simulink model "Zencar_rpo_2020_LQG_simModel_reactionWheel"  (R2020a)
settings: Solver=FixedStepAuto  StartTime=0.0  StopTime=40  FixedStep=1e-2  RelTol=1e-3
values from neighbouring files (symbols this model uses):
  A = a    [Zencar_rpo_2020_LQG_runScript_reactionWheel.m]    (also in Zencar_rpo_2020_LQG_simulationdata_reactionWheel.mat = [0  1  0; 21.2662842878  -0.985371341296  0.492685670648; -2)
  Ad = sysd.A    [Zencar_rpo_2020_LQG_runScript_reactionWheel.m]    (also in Zencar_rpo_2020_LQG_simulationdata_reactionWheel.mat = [1.00105829554  0.0099544956971  2.42643093775e-05; 0.211179)
  B = b    [Zencar_rpo_2020_LQG_runScript_reactionWheel.m]    (also in Zencar_rpo_2020_LQG_simulationdata_reactionWheel.mat = [0 -9.85371341296 72.353713413])
  Bd = sysd.B    [Zencar_rpo_2020_LQG_runScript_reactionWheel.m]    (also in Zencar_rpo_2020_LQG_simulationdata_reactionWheel.mat = [-0.00048528618755 -0.0963331348828 0.710167659151])
  bm = 0.05    [Zencar_rpo_2020_LQG_runScript_reactionWheel.m]    (also in Zencar_rpo_2020_LQG_simulationdata_reactionWheel.mat)
  bw = 0.1    [Zencar_rpo_2020_LQG_runScript_reactionWheel.m]    (also in Zencar_rpo_2020_LQG_simulationdata_reactionWheel.mat)
  C = c    [Zencar_rpo_2020_LQG_runScript_reactionWheel.m]    (also in Zencar_rpo_2020_LQG_simulationdata_reactionWheel.mat = [1  0  0; 0  1  0; 0  0  1])
  fi0 = -0.20    (= -0.2)    [Zencar_rpo_2020_LQG_runScript_reactionWheel.m]    (also in Zencar_rpo_2020_LQG_simulationdata_reactionWheel.mat)
  H = [1 0 0]    [Zencar_rpo_2020_LQG_runScript_reactionWheel.m]    (also in Zencar_rpo_2020_LQG_simulationdata_reactionWheel.mat)
  I = Imo+Iwo+Ibo    (= 0.101484583333)    [Zencar_rpo_2020_LQG_runScript_reactionWheel.m]    (also in Zencar_rpo_2020_LQG_simulationdata_reactionWheel.mat)
  Iw = mw*rw^2    (= 0.016)    [Zencar_rpo_2020_LQG_runScript_reactionWheel.m]    (also in Zencar_rpo_2020_LQG_simulationdata_reactionWheel.mat)
  K = k    [Zencar_rpo_2020_LQG_runScript_reactionWheel.m]    (also in Zencar_rpo_2020_LQG_simulationdata_reactionWheel.mat = [-13.1563542739 -3.87745747871 -0.104772255751])
  Kmgl = (mm*lm + mw*mw + mb*lb)*g    (= 2.1582)    [Zencar_rpo_2020_LQG_runScript_reactionWheel.m]    (also in Zencar_rpo_2020_LQG_simulationdata_reactionWheel.mat)
  P = zeros(3)    [Zencar_rpo_2020_LQG_runScript_reactionWheel.m]    (also in Zencar_rpo_2020_LQG_simulationdata_reactionWheel.mat = [0  0  0; 0  0  0; 0  0  0])
  V = 1*eye(3)    [Zencar_rpo_2020_LQG_runScript_reactionWheel.m]    (also in Zencar_rpo_2020_LQG_simulationdata_reactionWheel.mat = [1  0  0; 0  1  0; 0  0  1])
  W = 100    [Zencar_rpo_2020_LQG_runScript_reactionWheel.m]    (also in Zencar_rpo_2020_LQG_simulationdata_reactionWheel.mat)
  xhat = [fi0+(-1)^randi(10)*rand*2*pi/3200,0,0]'    [Zencar_rpo_2020_LQG_runScript_reactionWheel.m]    (also in Zencar_rpo_2020_LQG_simulationdata_reactionWheel.mat = [-0.200499281891 0 0])
undefined symbols (not defined in the file or in its folder): Continuous, Time
libraries: ctrlSharedLib x1
settings Model: Creator=Palo  LastModifiedBy=Palo
settings SolverCC: PositivePriorityOrder=on
settings DebuggingCC: InheritedTsInSrcMsg=none

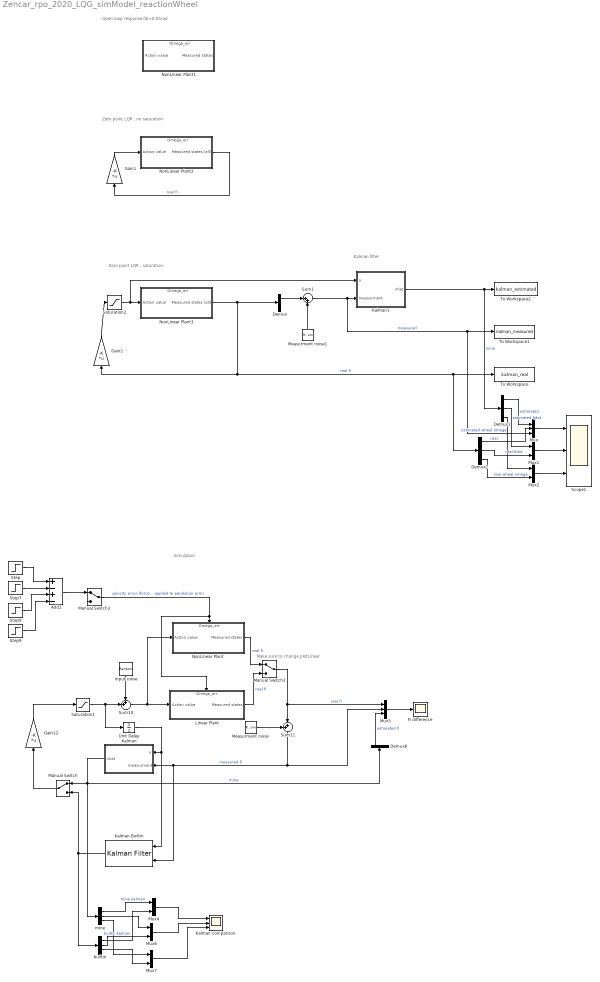
== system Zencar_rpo_2020_LQG_simModel_reactionWheel ==
  note: Open loop response fi0=0.05rad
  note: Zero point LQR , no saturation
  note: Zero point LQR , saturation
  note: Kalman filter
  note: Simulation
  note: Make sure to change plotLinear
  Add2 : Sum  Inputs=+-+-
  Demux{,1..2,6} (4 alike) : Demux  Outputs=3
  Fi difference : Scope
  Gain1 : Gain  Gain=-K  Multiplication=Matrix(K*u) (u vector)
  Gain12 : Gain  Gain=-K  Multiplication=Matrix(K*u) (u vector)
  Gain2 : Gain  Gain=-K  Multiplication=Matrix(K*u) (u vector)
  Input noise : RandomNumber  Variance=0.005  SampleTime=1e-2
  Kalman : Subsystem
  Kalman Builtin : ctrlSharedLib/Kalman Filter  TimeDomain=Continuous-Time  UseCurrentEstimator=on  ModelSource=Individual A, B, C, D matrices  ModelSourceVariable=sys  A=A  B=B  C=H  D=[0]  NumberOfStates=2  NumberOfInputs=2  NumberOfOutputs=2  InitialEstimateSource=Dialog  X0=xhat  P0=10  UseK=off  UseGH=off  NumberOfProcessNoiseInputs=2  G=1  TimeInvariantG=on  H=0  TimeInvariantH=on  Q=V  TimeInvariantQ=on  R=W  TimeInvariantR=on  N=0  TimeInvariantN=on  AddInputPort=on  AddEnablePort=off  OutputEstimatedY=off  OutputP=off  Ts=-1
  Kalman comparison : Scope  NumInputPorts=3
  Kalman1 : Subsystem
  Linear Plant : Subsystem
      settings: PortSchema="{\"entries\":[{\"content\":{\"sides\":[{\"content\":{\"connectorIds\":[\"In1\"]},\"type\":\"ConnectorPlacement.EquallySpacedRectSide\",\"uuid\":\"cef5a7e4-1169-406f-b141-8375d8af5010\"},{\"content\":{\"connectorIds\":[\"Out1\"],\"side\":\"RIGHT\"},\"type\":\"ConnectorPlacement.EquallySpacedRectSide\",\"uuid\":\"2cc08554-135f-4c1e-bb7d-3e74a7023c76\"},{\"content\":{\"connectorIds\":[\"In2\"],\"side\":\"TOP\"},\"type\":\"ConnectorPlacement.EquallySpacedRectSide\",\"uuid\":\"582a160d-15c5-42e8-87fa-6e353e2a7fa0\"}]},\"type\":\"ConnectorPlacement.EquallySpacedConnector\",\"uuid\":\"6957a99b-b85f-4d62-b482-e6d5ad956caf\"}],\"packageUris\":[\"http://schema.mathworks.com/mf0/Connector/19700101\"],\"version\":\"1.0\"}"
  Manual Switch : ManualSwitch
  Manual Switch2 : ManualSwitch
  Manual Switch3 : ManualSwitch
  Measurment noise : RandomNumber  Variance=2*pi/3200  SampleTime=1e-2
  Measurment noise1 : RandomNumber  Variance=2*pi/3200  SampleTime=1e-2
  Mux : Mux  Inputs=3
  Mux{1..2,4,6..7} (5 alike) : Mux  Inputs=2
  Mux5 : Mux  Inputs=3
  NonLinear Plant : Subsystem
      settings: PortSchema="{\"entries\":[{\"content\":{\"sides\":[{\"content\":{\"connectorIds\":[\"In1\"]},\"type\":\"ConnectorPlacement.EquallySpacedRectSide\",\"uuid\":\"cef5a7e4-1169-406f-b141-8375d8af5010\"},{\"content\":{\"connectorIds\":[\"Out1\"],\"side\":\"RIGHT\"},\"type\":\"ConnectorPlacement.EquallySpacedRectSide\",\"uuid\":\"2cc08554-135f-4c1e-bb7d-3e74a7023c76\"},{\"content\":{\"connectorIds\":[\"In2\"],\"side\":\"TOP\"},\"type\":\"ConnectorPlacement.EquallySpacedRectSide\",\"uuid\":\"582a160d-15c5-42e8-87fa-6e353e2a7fa0\"},{\"content\":{\"connectorIds\":[],\"side\":\"BOTTOM\"},\"type\":\"ConnectorPlacement.EquallySpacedRectSide\",\"uuid\":\"8b1cd8be-bae2-40ab-822a-6c2014c2b0d3\"}]},\"type\":\"ConnectorPlacement.EquallySpacedConnector\",\"uuid\":\"6957a99b-b85f-4d62-b482-e6d5ad956caf\"}],\"packageUris\":[\"http://schema.mathworks.com/mf0/Connector/19700101\"],\"version\":\"1.0\"}"
  NonLinear Plant1 : Subsystem
      settings: PortSchema="{\"entries\":[{\"content\":{\"sides\":[{\"content\":{\"connectorIds\":[\"In1\"]},\"type\":\"ConnectorPlacement.EquallySpacedRectSide\",\"uuid\":\"cef5a7e4-1169-406f-b141-8375d8af5010\"},{\"content\":{\"connectorIds\":[\"Out1\"],\"side\":\"RIGHT\"},\"type\":\"ConnectorPlacement.EquallySpacedRectSide\",\"uuid\":\"2cc08554-135f-4c1e-bb7d-3e74a7023c76\"},{\"content\":{\"connectorIds\":[\"In2\"],\"side\":\"TOP\"},\"type\":\"ConnectorPlacement.EquallySpacedRectSide\",\"uuid\":\"582a160d-15c5-42e8-87fa-6e353e2a7fa0\"},{\"content\":{\"connectorIds\":[],\"side\":\"BOTTOM\"},\"type\":\"ConnectorPlacement.EquallySpacedRectSide\",\"uuid\":\"8b1cd8be-bae2-40ab-822a-6c2014c2b0d3\"}]},\"type\":\"ConnectorPlacement.EquallySpacedConnector\",\"uuid\":\"6957a99b-b85f-4d62-b482-e6d5ad956caf\"}],\"packageUris\":[\"http://schema.mathworks.com/mf0/Connector/19700101\"],\"version\":\"1.0\"}"
  NonLinear Plant2 : Subsystem
      settings: PortSchema="{\"entries\":[{\"content\":{\"sides\":[{\"content\":{\"connectorIds\":[\"In1\"]},\"type\":\"ConnectorPlacement.EquallySpacedRectSide\",\"uuid\":\"cef5a7e4-1169-406f-b141-8375d8af5010\"},{\"content\":{\"connectorIds\":[\"Out1\"],\"side\":\"RIGHT\"},\"type\":\"ConnectorPlacement.EquallySpacedRectSide\",\"uuid\":\"2cc08554-135f-4c1e-bb7d-3e74a7023c76\"},{\"content\":{\"connectorIds\":[\"In2\"],\"side\":\"TOP\"},\"type\":\"ConnectorPlacement.EquallySpacedRectSide\",\"uuid\":\"582a160d-15c5-42e8-87fa-6e353e2a7fa0\"},{\"content\":{\"connectorIds\":[],\"side\":\"BOTTOM\"},\"type\":\"ConnectorPlacement.EquallySpacedRectSide\",\"uuid\":\"8b1cd8be-bae2-40ab-822a-6c2014c2b0d3\"}]},\"type\":\"ConnectorPlacement.EquallySpacedConnector\",\"uuid\":\"6957a99b-b85f-4d62-b482-e6d5ad956caf\"}],\"packageUris\":[\"http://schema.mathworks.com/mf0/Connector/19700101\"],\"version\":\"1.0\"}"
  NonLinear Plant3 : Subsystem
      settings: PortSchema="{\"entries\":[{\"content\":{\"sides\":[{\"content\":{\"connectorIds\":[\"In1\"]},\"type\":\"ConnectorPlacement.EquallySpacedRectSide\",\"uuid\":\"cef5a7e4-1169-406f-b141-8375d8af5010\"},{\"content\":{\"connectorIds\":[\"Out1\"],\"side\":\"RIGHT\"},\"type\":\"ConnectorPlacement.EquallySpacedRectSide\",\"uuid\":\"2cc08554-135f-4c1e-bb7d-3e74a7023c76\"},{\"content\":{\"connectorIds\":[\"In2\"],\"side\":\"TOP\"},\"type\":\"ConnectorPlacement.EquallySpacedRectSide\",\"uuid\":\"582a160d-15c5-42e8-87fa-6e353e2a7fa0\"},{\"content\":{\"connectorIds\":[],\"side\":\"BOTTOM\"},\"type\":\"ConnectorPlacement.EquallySpacedRectSide\",\"uuid\":\"8b1cd8be-bae2-40ab-822a-6c2014c2b0d3\"}]},\"type\":\"ConnectorPlacement.EquallySpacedConnector\",\"uuid\":\"6957a99b-b85f-4d62-b482-e6d5ad956caf\"}],\"packageUris\":[\"http://schema.mathworks.com/mf0/Connector/19700101\"],\"version\":\"1.0\"}"
  Saturation1 : Saturate  UpperLimit=0.8  LowerLimit=-0.8
  Saturation2 : Saturate  UpperLimit=0.8  LowerLimit=-0.8
  Scope1 : Scope  NumInputPorts=3
  Step : Step  Time=3  After=4  SampleTime=0
  Step7 : Step  Time=3.05  After=4  SampleTime=0
  Step8 : Step  Time=5.6  After=-4  SampleTime=0
  Step9 : Step  Time=5.65  After=-4  SampleTime=0
  Sum1 : Sum  Inputs=|++
  Sum10 : Sum  Inputs=++|
  Sum11 : Sum  Inputs=++|
  To Workspace : ToWorkspace  VariableName=kalman_real  SaveFormat=Structure With Time  SampleTime=-1
  To Workspace1 : ToWorkspace  VariableName=kalman_measured  SaveFormat=Structure With Time  SampleTime=-1
  To Workspace2 : ToWorkspace  VariableName=kalman_estimated  SaveFormat=Structure With Time  SampleTime=-1
  Unit Delay : UnitDelay  SampleTime=-1  HasFrameUpgradeWarning=on
  builtin : Demux  Outputs=3
  mine : Demux  Outputs=3
  wires:
  Mux5/1 -> Fi difference/1
  Saturation1/1 -> Unit Delay/1, Sum10/2
  Kalman/1(xhat) -> Demux6/1, Manual Switch/1, mine/1  "mine"
  Kalman Builtin/1 -> Manual Switch/2, builtin/1
  Sum11/1 -> Mux5/2, Kalman Builtin/2, Kalman/2(measurment)  "measured fi"
  Demux6/1 -> Mux5/3  "estimated fi"
  Linear Plant/1(Measured states) -> Manual Switch2/2  "real fi"
  NonLinear Plant/1(Measured states) -> Manual Switch2/1  "real fi"
  Manual Switch2/1 -> Mux5/1, Sum11/2  "real fi"
  Step/1 -> Add2/1
  Step7/1 -> Add2/2
  Step8/1 -> Add2/3
  Step9/1 -> Add2/4
  Manual Switch3/1 -> Linear Plant/2(Omega_err), NonLinear Plant/2(Omega_err)  "velocity error (force applied to pendulum arm)"
  Add2/1 -> Manual Switch3/1
  Sum10/1 -> NonLinear Plant/1(Action value), Linear Plant/1(Action value)
  mine/1 -> Mux4/1  "mine kalman"
  builtin/1 -> Mux4/2  "builtin kalman"
  mine/2 -> Mux6/1
  mine/3 -> Mux7/1
  builtin/2 -> Mux6/2
  builtin/3 -> Mux7/2
  Mux4/1 -> Kalman comparison/1
  Mux6/1 -> Kalman comparison/2
  Mux7/1 -> Kalman comparison/3
  Unit Delay/1 -> Kalman Builtin/1, Kalman/1(u)
  Gain12/1 -> Saturation1/1
  Manual Switch/1 -> Gain12/1
  NonLinear Plant2/1(Measured states (all)) -> Gain1/1  "real fi"
  Gain1/1 -> NonLinear Plant2/1(Action value)
  Measurment noise/1 -> Sum11/1
  Gain2/1 -> Saturation2/1
  NonLinear Plant3/1(Measured states (all)) -> Demux/1, Gain2/1, Demux2/1, To Workspace/1  "real fi"
  Saturation2/1 -> Kalman1/1(u), NonLinear Plant3/1(Action value)
  Measurment noise1/1 -> Sum1/2
  Demux/1 -> Sum1/1
  Sum1/1 -> To Workspace1/1, Mux/3, Kalman1/2(measurment)  "measured"
  Kalman1/1(xhat) -> Demux1/1, To Workspace2/1  "mine"
  Mux/1 -> Scope1/1
  Mux1/1 -> Scope1/2
  Mux2/1 -> Scope1/3
  Demux1/1 -> Mux/1  "estimated"
  Demux1/2 -> Mux1/1  "estimated fidot"
  Demux1/3 -> Mux2/1  "estimated wheel omega"
  Demux2/1 -> Mux/2  "real"
  Demux2/2 -> Mux1/2  "real fidot"
  Demux2/3 -> Mux2/2  "real wheel omega"
  Input noise/1 -> Sum10/1

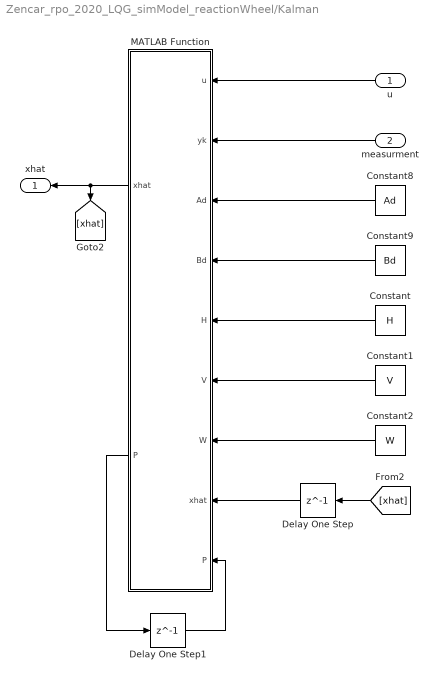
== system Zencar_rpo_2020_LQG_simModel_reactionWheel/Kalman ==
  u : Inport
  measurment : Inport  Port=2
  Constant : Constant  Value=H  VectorParams1D=off
  Constant1 : Constant  Value=V  VectorParams1D=off
  Constant2 : Constant  Value=W  VectorParams1D=off
  Constant8 : Constant  Value=Ad  VectorParams1D=off
  Constant9 : Constant  Value=Bd  VectorParams1D=off
  Delay One Step : Delay  DelayLength=1  InitialCondition=xhat
  Delay One Step1 : Delay  DelayLength=1  InitialCondition=P
  MATLAB Function : MATLAB Function  TreatAsAtomicUnit=on
  xhat : Outport
  wires:
  Delay One Step/1 -> MATLAB Function/8("xhat ")
  MATLAB Function/1(xhat) -> xhat/1, [xhat]
  MATLAB Function/2(P) -> Delay One Step1/1
  [xhat] -> Delay One Step/1
  measurment/1 -> MATLAB Function/2(yk)
  u/1 -> MATLAB Function/1(u)
  Delay One Step1/1 -> MATLAB Function/9("P ")
  Constant2/1 -> MATLAB Function/7(W)
  Constant1/1 -> MATLAB Function/6(V)
  Constant/1 -> MATLAB Function/5(H)
  Constant9/1 -> MATLAB Function/4(Bd)
  Constant8/1 -> MATLAB Function/3(Ad)

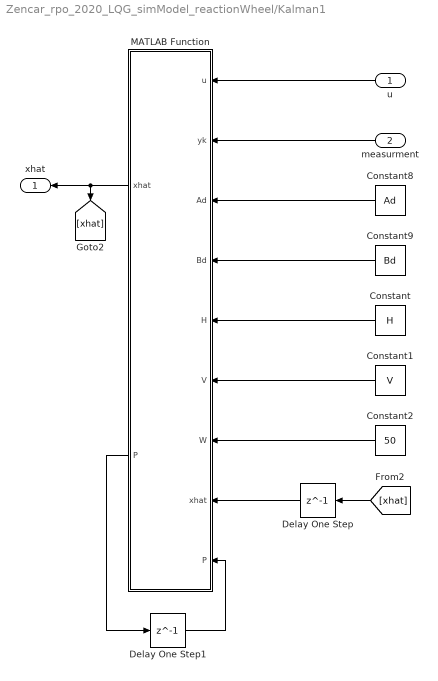
== system Zencar_rpo_2020_LQG_simModel_reactionWheel/Kalman1 ==
  u : Inport
  measurment : Inport  Port=2
  Constant : Constant  Value=H  VectorParams1D=off
  Constant1 : Constant  Value=V  VectorParams1D=off
  Constant2 : Constant  Value=50  VectorParams1D=off
  Constant8 : Constant  Value=Ad  VectorParams1D=off
  Constant9 : Constant  Value=Bd  VectorParams1D=off
  Delay One Step : Delay  DelayLength=1  InitialCondition=[0.2,0,0]'
  Delay One Step1 : Delay  DelayLength=1  InitialCondition=P
  MATLAB Function : MATLAB Function  TreatAsAtomicUnit=on
  xhat : Outport
  wires:
  Constant8/1 -> MATLAB Function/3(Ad)
  Constant9/1 -> MATLAB Function/4(Bd)
  Constant/1 -> MATLAB Function/5(H)
  Constant1/1 -> MATLAB Function/6(V)
  Constant2/1 -> MATLAB Function/7(W)
  Delay One Step1/1 -> MATLAB Function/9("P ")
  u/1 -> MATLAB Function/1(u)
  measurment/1 -> MATLAB Function/2(yk)
  [xhat] -> Delay One Step/1
  MATLAB Function/2(P) -> Delay One Step1/1
  MATLAB Function/1(xhat) -> [xhat], xhat/1
  Delay One Step/1 -> MATLAB Function/8("xhat ")

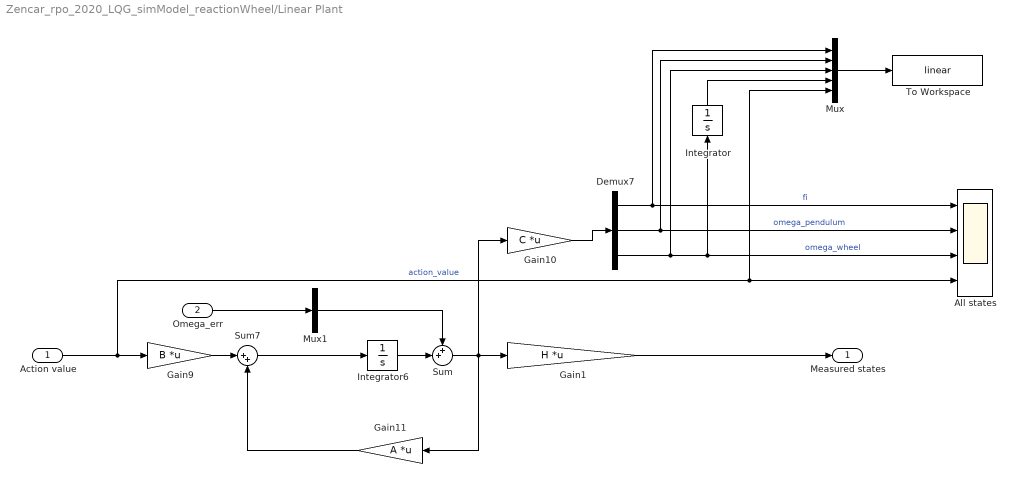
== system Zencar_rpo_2020_LQG_simModel_reactionWheel/Linear Plant ==
  Action value : Inport
  Omega_err : Inport  Port=2
  All states : Scope  NumInputPorts=4
  Demux7 : Demux  Outputs=3
  Gain1 : Gain  Gain=H  Multiplication=Matrix(K*u) (u vector)
  Gain10 : Gain  Gain=C  Multiplication=Matrix(K*u) (u vector)
  Gain11 : Gain  Gain=A  Multiplication=Matrix(K*u) (u vector)
  Gain9 : Gain  Gain=B  Multiplication=Matrix(K*u) (u vector)
  Integrator : Integrator
  Integrator6 : Integrator  InitialCondition=[fi0;0;0]
  Mux : Mux  Inputs=5
  Mux1 : Mux  Inputs=3
  Sum : Sum  Inputs=++|
  Sum7 : Sum  Inputs=|++
  To Workspace : ToWorkspace  VariableName=linear  SaveFormat=Structure With Time  SampleTime=-1
  Measured states : Outport
  wires:
  Gain9/1 -> Sum7/1
  Demux7/2 -> Mux/2, All states/2  "omega_pendulum"
  Demux7/3 -> Mux/3, Integrator/1, All states/3  "omega_wheel"
  Demux7/1 -> Mux/1, All states/1  "fi"
  Gain10/1 -> Demux7/1
  Gain11/1 -> Sum7/2
  Sum7/1 -> Integrator6/1
  Gain1/1 -> Measured states/1
  Action value/1 -> Mux/5, All states/4, Gain9/1  "action_value"
  Mux/1 -> To Workspace/1
  Integrator/1 -> Mux/4
  Omega_err/1 -> Mux1/2
  Mux1/1 -> Sum/1
  Integrator6/1 -> Sum/2
  Sum/1 -> Gain10/1, Gain11/1, Gain1/1

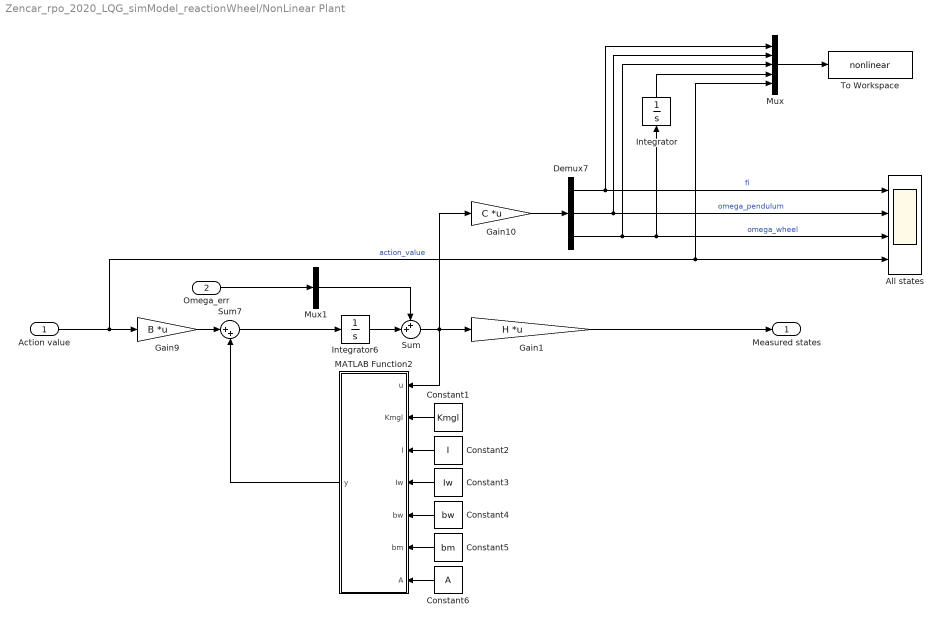
== system Zencar_rpo_2020_LQG_simModel_reactionWheel/NonLinear Plant ==
  Action value : Inport
  Omega_err : Inport  Port=2
  All states : Scope  NumInputPorts=4
  Constant1 : Constant  Value=Kmgl
  Constant2 : Constant  Value=I
  Constant3 : Constant  Value=Iw
  Constant4 : Constant  Value=bw
  Constant5 : Constant  Value=bm
  Constant6 : Constant  Value=A
  Demux7 : Demux  Outputs=3
  Gain1 : Gain  Gain=H  Multiplication=Matrix(K*u) (u vector)
  Gain10 : Gain  Gain=C  Multiplication=Matrix(K*u) (u vector)
  Gain9 : Gain  Gain=B  Multiplication=Matrix(K*u) (u vector)
  Integrator : Integrator
  Integrator6 : Integrator  InitialCondition=[fi0;0;0]
  MATLAB Function2 : MATLAB Function  TreatAsAtomicUnit=on
  Mux : Mux  Inputs=5
  Mux1 : Mux  Inputs=3
  Sum : Sum  Inputs=++|
  Sum7 : Sum  Inputs=|++
  To Workspace : ToWorkspace  VariableName=nonlinear  SaveFormat=Structure With Time  SampleTime=-1
  Measured states : Outport
  wires:
  Gain9/1 -> Sum7/1
  Demux7/2 -> Mux/2, All states/2  "omega_pendulum"
  Demux7/3 -> Mux/3, Integrator/1, All states/3  "omega_wheel"
  Demux7/1 -> Mux/1, All states/1  "fi"
  Gain10/1 -> Demux7/1
  Sum7/1 -> Integrator6/1
  Action value/1 -> Mux/5, All states/4, Gain9/1  "action_value"
  Mux/1 -> To Workspace/1
  Integrator/1 -> Mux/4
  Constant4/1 -> MATLAB Function2/5(bw)
  Constant3/1 -> MATLAB Function2/4(Iw)
  Constant5/1 -> MATLAB Function2/6(bm)
  Constant1/1 -> MATLAB Function2/2(Kmgl)
  MATLAB Function2/1(y) -> Sum7/2
  Constant2/1 -> MATLAB Function2/3(I)
  Integrator6/1 -> Sum/2
  Sum/1 -> Gain10/1, MATLAB Function2/1(u), Gain1/1
  Mux1/1 -> Sum/1
  Omega_err/1 -> Mux1/2
  Gain1/1 -> Measured states/1
  Constant6/1 -> MATLAB Function2/7(A)

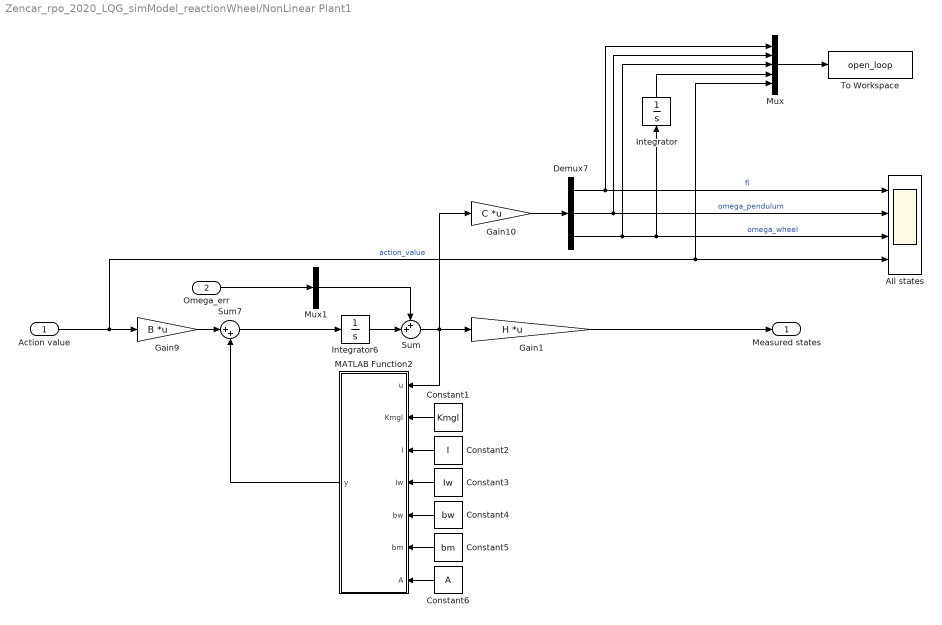
== system Zencar_rpo_2020_LQG_simModel_reactionWheel/NonLinear Plant1 ==
  Action value : Inport
  Omega_err : Inport  Port=2
  All states : Scope  NumInputPorts=4
  Constant1 : Constant  Value=Kmgl
  Constant2 : Constant  Value=I
  Constant3 : Constant  Value=Iw
  Constant4 : Constant  Value=bw
  Constant5 : Constant  Value=bm
  Constant6 : Constant  Value=A
  Demux7 : Demux  Outputs=3
  Gain1 : Gain  Gain=H  Multiplication=Matrix(K*u) (u vector)
  Gain10 : Gain  Gain=C  Multiplication=Matrix(K*u) (u vector)
  Gain9 : Gain  Gain=B  Multiplication=Matrix(K*u) (u vector)
  Integrator : Integrator
  Integrator6 : Integrator  InitialCondition=[0.05;0;0]
  MATLAB Function2 : MATLAB Function  TreatAsAtomicUnit=on
  Mux : Mux  Inputs=5
  Mux1 : Mux  Inputs=3
  Sum : Sum  Inputs=++|
  Sum7 : Sum  Inputs=|++
  To Workspace : ToWorkspace  VariableName=open_loop  SaveFormat=Structure With Time  SampleTime=-1
  Measured states : Outport
  wires:
  Constant6/1 -> MATLAB Function2/7(A)
  Gain1/1 -> Measured states/1
  Omega_err/1 -> Mux1/2
  Mux1/1 -> Sum/1
  Sum/1 -> Gain1/1, MATLAB Function2/1(u), Gain10/1
  Integrator6/1 -> Sum/2
  Constant2/1 -> MATLAB Function2/3(I)
  MATLAB Function2/1(y) -> Sum7/2
  Constant1/1 -> MATLAB Function2/2(Kmgl)
  Constant5/1 -> MATLAB Function2/6(bm)
  Constant3/1 -> MATLAB Function2/4(Iw)
  Constant4/1 -> MATLAB Function2/5(bw)
  Integrator/1 -> Mux/4
  Mux/1 -> To Workspace/1
  Action value/1 -> Gain9/1, All states/4, Mux/5  "action_value"
  Sum7/1 -> Integrator6/1
  Gain10/1 -> Demux7/1
  Demux7/1 -> All states/1, Mux/1  "fi"
  Demux7/3 -> All states/3, Integrator/1, Mux/3  "omega_wheel"
  Demux7/2 -> All states/2, Mux/2  "omega_pendulum"
  Gain9/1 -> Sum7/1

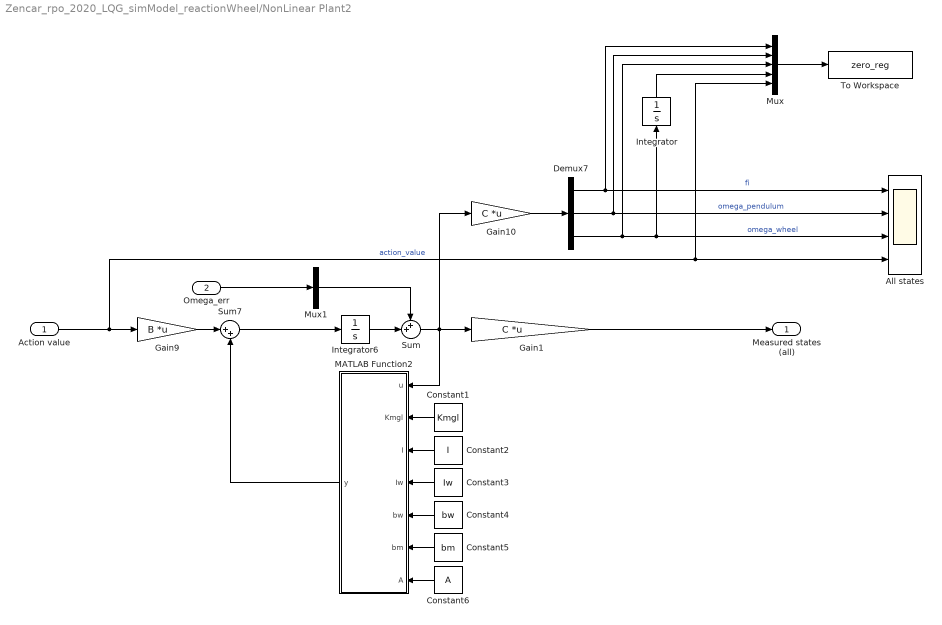
== system Zencar_rpo_2020_LQG_simModel_reactionWheel/NonLinear Plant2 ==
  Action value : Inport
  Omega_err : Inport  Port=2
  All states : Scope  NumInputPorts=4
  Constant1 : Constant  Value=Kmgl
  Constant2 : Constant  Value=I
  Constant3 : Constant  Value=Iw
  Constant4 : Constant  Value=bw
  Constant5 : Constant  Value=bm
  Constant6 : Constant  Value=A
  Demux7 : Demux  Outputs=3
  Gain1 : Gain  Gain=C  Multiplication=Matrix(K*u) (u vector)
  Gain10 : Gain  Gain=C  Multiplication=Matrix(K*u) (u vector)
  Gain9 : Gain  Gain=B  Multiplication=Matrix(K*u) (u vector)
  Integrator : Integrator
  Integrator6 : Integrator  InitialCondition=[-0.2;0;0]
  MATLAB Function2 : MATLAB Function  TreatAsAtomicUnit=on
  Mux : Mux  Inputs=5
  Mux1 : Mux  Inputs=3
  Sum : Sum  Inputs=++|
  Sum7 : Sum  Inputs=|++
  To Workspace : ToWorkspace  VariableName=zero_reg  SaveFormat=Structure With Time  SampleTime=-1
  Measured states (all) : Outport
  wires:
  Constant6/1 -> MATLAB Function2/7(A)
  Gain1/1 -> Measured states (all)/1
  Omega_err/1 -> Mux1/2
  Mux1/1 -> Sum/1
  Sum/1 -> Gain1/1, MATLAB Function2/1(u), Gain10/1
  Integrator6/1 -> Sum/2
  Constant2/1 -> MATLAB Function2/3(I)
  MATLAB Function2/1(y) -> Sum7/2
  Constant1/1 -> MATLAB Function2/2(Kmgl)
  Constant5/1 -> MATLAB Function2/6(bm)
  Constant3/1 -> MATLAB Function2/4(Iw)
  Constant4/1 -> MATLAB Function2/5(bw)
  Integrator/1 -> Mux/4
  Mux/1 -> To Workspace/1
  Action value/1 -> Gain9/1, All states/4, Mux/5  "action_value"
  Sum7/1 -> Integrator6/1
  Gain10/1 -> Demux7/1
  Demux7/1 -> All states/1, Mux/1  "fi"
  Demux7/3 -> All states/3, Integrator/1, Mux/3  "omega_wheel"
  Demux7/2 -> All states/2, Mux/2  "omega_pendulum"
  Gain9/1 -> Sum7/1

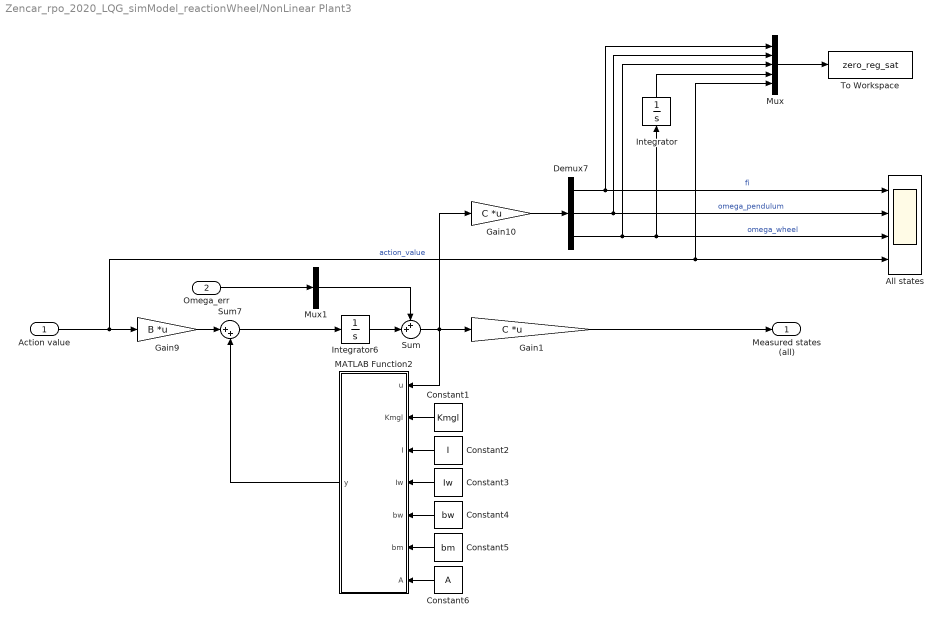
== system Zencar_rpo_2020_LQG_simModel_reactionWheel/NonLinear Plant3 ==
  Action value : Inport
  Omega_err : Inport  Port=2
  All states : Scope  NumInputPorts=4
  Constant1 : Constant  Value=Kmgl
  Constant2 : Constant  Value=I
  Constant3 : Constant  Value=Iw
  Constant4 : Constant  Value=bw
  Constant5 : Constant  Value=bm
  Constant6 : Constant  Value=A
  Demux7 : Demux  Outputs=3
  Gain1 : Gain  Gain=C  Multiplication=Matrix(K*u) (u vector)
  Gain10 : Gain  Gain=C  Multiplication=Matrix(K*u) (u vector)
  Gain9 : Gain  Gain=B  Multiplication=Matrix(K*u) (u vector)
  Integrator : Integrator
  Integrator6 : Integrator  InitialCondition=[-0.2;0;0]
  MATLAB Function2 : MATLAB Function  TreatAsAtomicUnit=on
  Mux : Mux  Inputs=5
  Mux1 : Mux  Inputs=3
  Sum : Sum  Inputs=++|
  Sum7 : Sum  Inputs=|++
  To Workspace : ToWorkspace  VariableName=zero_reg_sat  SaveFormat=Structure With Time  SampleTime=-1
  Measured states (all) : Outport
  wires:
  Constant6/1 -> MATLAB Function2/7(A)
  Gain1/1 -> Measured states (all)/1
  Omega_err/1 -> Mux1/2
  Mux1/1 -> Sum/1
  Sum/1 -> Gain1/1, MATLAB Function2/1(u), Gain10/1
  Integrator6/1 -> Sum/2
  Constant2/1 -> MATLAB Function2/3(I)
  MATLAB Function2/1(y) -> Sum7/2
  Constant1/1 -> MATLAB Function2/2(Kmgl)
  Constant5/1 -> MATLAB Function2/6(bm)
  Constant3/1 -> MATLAB Function2/4(Iw)
  Constant4/1 -> MATLAB Function2/5(bw)
  Integrator/1 -> Mux/4
  Mux/1 -> To Workspace/1
  Action value/1 -> Gain9/1, All states/4, Mux/5  "action_value"
  Sum7/1 -> Integrator6/1
  Gain10/1 -> Demux7/1
  Demux7/1 -> All states/1, Mux/1  "fi"
  Demux7/3 -> All states/3, Integrator/1, Mux/3  "omega_wheel"
  Demux7/2 -> All states/2, Mux/2  "omega_pendulum"
  Gain9/1 -> Sum7/1

== matlab function Zencar_rpo_2020_LQG_simModel_reactionWheel/NonLinear Plant/MATLAB Function2 ==
  data: u input; y output; Kmgl input; I input; Iw input; bw input; bm input; A input
function y = fcn(u,Kmgl,I,Iw,bw,bm,A)
y=[0;0;0];
% 
% y(1)=u(2);
% y(2)=+(Kmgl/(I-Iw))*sin(u(1)) - (bw/(I-Iw))*u(2) + (bm*Iw/(I-Iw))*u(3);
% y(3)=-(Kmgl/I/(1-(Iw/I)))*sin(u(1)) + (bw/I/(1-(Iw/I)))*u(2) - (bm/I/(1-(Iw/I)))*u(3);


y(1)=A(1,1)*u(1)+A(1,2)*u(2)+A(1,3)*u(3);
y(2)=A(2,1)*sin(u(1))+A(2,2)*u(2)+A(2,3)*u(3);
y(3)=A(3,1)*sin(u(1))+A(3,2)*u(2)+A(3,3)*u(3);

== matlab function Zencar_rpo_2020_LQG_simModel_reactionWheel/Kalman/MATLAB Function ==
  data: u input; yk input; xhat output; P output; Ad input; Bd input; H input; V input; W input; xhat input; P input
function [xhat,P] = fcn(u,yk,Ad,Bd,H,V,W,xhat,P)


    xhatk1k=Ad*xhat+Bd*u;
    Pk1k=Ad*P*Ad'+V;

    yhat=H*xhatk1k;
    ywave=yk-yhat;
    S=H*Pk1k*H' + W;
    K=P*H'*inv(S);
    
    xhatk1k1=xhatk1k+K*ywave;
    %Pk1k1=Pk1k-K*S*K';
    Pk1k1=(eye(3)-K*H)*Pk1k;
    
    xhat=xhatk1k1;
    P=Pk1k1;

    


end

== matlab function Zencar_rpo_2020_LQG_simModel_reactionWheel/NonLinear Plant1/MATLAB Function2 ==
  data: u input; y output; Kmgl input; I input; Iw input; bw input; bm input; A input
function y = fcn(u,Kmgl,I,Iw,bw,bm,A)
y=[0;0;0];
% 
% y(1)=u(2);
% y(2)=+(Kmgl/(I-Iw))*sin(u(1)) - (bw/(I-Iw))*u(2) + (bm*Iw/(I-Iw))*u(3);
% y(3)=-(Kmgl/I/(1-(Iw/I)))*sin(u(1)) + (bw/I/(1-(Iw/I)))*u(2) - (bm/I/(1-(Iw/I)))*u(3);


y(1)=A(1,1)*u(1)+A(1,2)*u(2)+A(1,3)*u(3);
y(2)=A(2,1)*sin(u(1))+A(2,2)*u(2)+A(2,3)*u(3);
y(3)=A(3,1)*sin(u(1))+A(3,2)*u(2)+A(3,3)*u(3);

== matlab function Zencar_rpo_2020_LQG_simModel_reactionWheel/NonLinear Plant2/MATLAB Function2 ==
  data: u input; y output; Kmgl input; I input; Iw input; bw input; bm input; A input
function y = fcn(u,Kmgl,I,Iw,bw,bm,A)
y=[0;0;0];
% 
% y(1)=u(2);
% y(2)=+(Kmgl/(I-Iw))*sin(u(1)) - (bw/(I-Iw))*u(2) + (bm*Iw/(I-Iw))*u(3);
% y(3)=-(Kmgl/I/(1-(Iw/I)))*sin(u(1)) + (bw/I/(1-(Iw/I)))*u(2) - (bm/I/(1-(Iw/I)))*u(3);


y(1)=A(1,1)*u(1)+A(1,2)*u(2)+A(1,3)*u(3);
y(2)=A(2,1)*sin(u(1))+A(2,2)*u(2)+A(2,3)*u(3);
y(3)=A(3,1)*sin(u(1))+A(3,2)*u(2)+A(3,3)*u(3);

== matlab function Zencar_rpo_2020_LQG_simModel_reactionWheel/NonLinear Plant3/MATLAB Function2 ==
  data: u input; y output; Kmgl input; I input; Iw input; bw input; bm input; A input
function y = fcn(u,Kmgl,I,Iw,bw,bm,A)
y=[0;0;0];
% 
% y(1)=u(2);
% y(2)=+(Kmgl/(I-Iw))*sin(u(1)) - (bw/(I-Iw))*u(2) + (bm*Iw/(I-Iw))*u(3);
% y(3)=-(Kmgl/I/(1-(Iw/I)))*sin(u(1)) + (bw/I/(1-(Iw/I)))*u(2) - (bm/I/(1-(Iw/I)))*u(3);


y(1)=A(1,1)*u(1)+A(1,2)*u(2)+A(1,3)*u(3);
y(2)=A(2,1)*sin(u(1))+A(2,2)*u(2)+A(2,3)*u(3);
y(3)=A(3,1)*sin(u(1))+A(3,2)*u(2)+A(3,3)*u(3);

== matlab function Zencar_rpo_2020_LQG_simModel_reactionWheel/Kalman1/MATLAB Function ==
  data: u input; yk input; xhat output; P output; Ad input; Bd input; H input; V input; W input; xhat input; P input
function [xhat,P] = fcn(u,yk,Ad,Bd,H,V,W,xhat,P)


    xhatk1k=Ad*xhat+Bd*u;
    Pk1k=Ad*P*Ad'+V;

    yhat=H*xhatk1k;
    ywave=yk-yhat;
    S=H*Pk1k*H' + W;
    K=P*H'*inv(S);
    
    xhatk1k1=xhatk1k+K*ywave;
    Pk1k1=(eye(3)-K*H)*Pk1k;
    
    xhat=xhatk1k1;
    P=Pk1k1;

   
end
